simulink model "ex3"  (R2019b)
settings: Solver=VariableStepAuto  StartTime=0.0  StopTime=10.0  RelTol=1e-3
undefined symbols (not defined in the file or in its folder): DiscIntNeverNeededParam
settings Model: Creator=samuelvenzi  LastModifiedBy=samuelvenzi

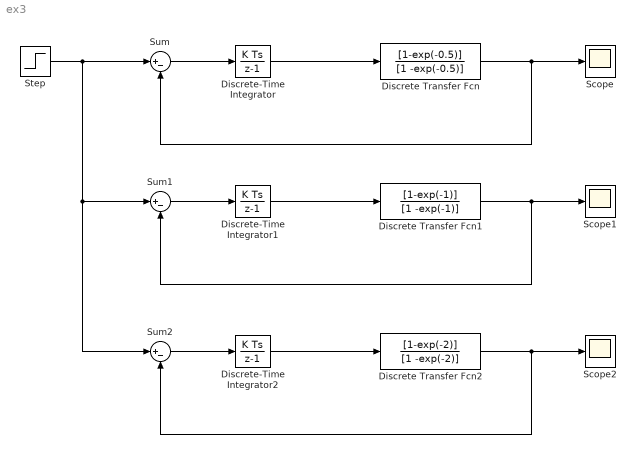
== system ex3 ==
  Discrete Transfer Fcn : DiscreteTransferFcn  Numerator=[1-exp(-0.5)]  Denominator=[1 -exp(-0.5)]
  Discrete Transfer Fcn1 : DiscreteTransferFcn  Numerator=[1-exp(-1)]  Denominator=[1 -exp(-1)]
  Discrete Transfer Fcn2 : DiscreteTransferFcn  Numerator=[1-exp(-2)]  Denominator=[1 -exp(-2)]
  Discrete-Time Integrator : DiscreteIntegrator  gainval=2  SampleTime=0.5  ICPrevOutput=DiscIntNeverNeededParam  ICPrevScaledInput=DiscIntNeverNeededParam
  Discrete-Time Integrator1 : DiscreteIntegrator  gainval=2  ICPrevOutput=DiscIntNeverNeededParam  ICPrevScaledInput=DiscIntNeverNeededParam
  Discrete-Time Integrator2 : DiscreteIntegrator  gainval=2  SampleTime=2  ICPrevOutput=DiscIntNeverNeededParam  ICPrevScaledInput=DiscIntNeverNeededParam
  Scope : Scope
  Scope1 : Scope
  Scope2 : Scope
  Step : Step  SampleTime=0
  Sum : Sum  Inputs=|+-
  Sum1 : Sum  Inputs=|+-
  Sum2 : Sum  Inputs=|+-
  wires:
  Discrete-Time Integrator/1 -> Discrete Transfer Fcn/1
  Sum/1 -> Discrete-Time Integrator/1
  Discrete Transfer Fcn/1 -> Sum/2, Scope/1
  Discrete Transfer Fcn1/1 -> Sum1/2, Scope1/1
  Discrete-Time Integrator1/1 -> Discrete Transfer Fcn1/1
  Sum1/1 -> Discrete-Time Integrator1/1
  Discrete Transfer Fcn2/1 -> Sum2/2, Scope2/1
  Step/1 -> Sum2/1, Sum1/1, Sum/1
  Discrete-Time Integrator2/1 -> Discrete Transfer Fcn2/1
  Sum2/1 -> Discrete-Time Integrator2/1
